simulink model "ex04_espeak"  (R2016a)
settings: Solver=FixedStepAuto  StartTime=0.0  StopTime=10.0  RelTol=1e-3
libraries: embdlinuxlib x1
settings Model: SimulationMode=external  Creator=ohori  LastModifiedBy=ohori
settings SolverCC: PositivePriorityOrder=on
settings OptimizationCC: OptimizeModelRefInitCode=on  LifeSpan=1  MaxStackSize=64
settings HardwareCC: ProdBitPerPointer=32  ProdLargestAtomicInteger=Long  ProdLargestAtomicFloat=Double  ProdWordSize=32  ProdHWDeviceType=ARM Compatible->ARM Cortex  UseEmbeddedCoderFeatures=off  UseSimulinkCoderFeatures=off
settings RTWCC: SystemTargetFile=ert.tlc  HardwareBoard=Raspberry Pi  TemplateMakefile=ert_default_tmf  GenerateReport=on  Toolchain=GNU GCC Raspberry Pi  IncludeHyperlinkInReport=on  LaunchReport=on  GenerateTraceInfo=on  GenerateTraceReport=on  GenerateTraceReportSl=on  GenerateTraceReportSf=on  GenerateTraceReportEml=on
settings CodeAppCC: ForceParamTrailComments=on  IgnoreCustomStorageClasses=off  OperatorAnnotations=on  SimulinkDataObjDesc=on  SFDataObjDesc=on  MATLABFcnDesc=on  InsertBlockDesc=on  MATLABSourceComments=on
settings ERTTargetCC: SupportNonInlinedSFcns=on  SupportVariableSizeSignals=on

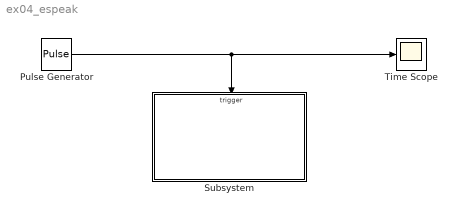
== system ex04_espeak ==
  Pulse Generator : DiscretePulseGenerator  Period=100  PulseWidth=5  SampleTime=0.1
  Subsystem : Subsystem
  Time Scope : Scope
  wires:
  Pulse Generator/1 -> Time Scope/1, Subsystem/Trigger

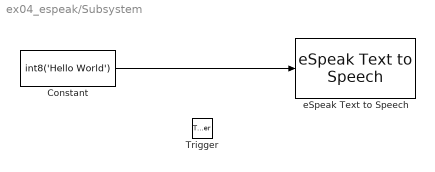
== system ex04_espeak/Subsystem ==
  Trigger : TriggerPort  TriggerType=falling  VariantControl=Variant  PortDimensions=1
  Constant : Constant  Value=int8('Hello World')
  eSpeak Text to Speech : embdlinuxlib/eSpeak Text to Speech  blockPlatform=Raspberry Pi
  wires:
  Constant/1 -> eSpeak Text to Speech/1
